simulink model "modi1_4"  (R2022b)
settings: Solver=VariableStepAuto  StartTime=0.0  StopTime=100.0  RelTol=1e-3
values from neighbouring files (symbols this model uses):
  a0 = 0.00447127    [modi1.m]
  a1 = 0.108205    [modi1.m]
  a2 = 0.683702    [modi1.m]
  alfa1 = 1.2    [modi1.m]
  alfa2 = 0.56    [modi1.m]
  alfa3 = -1.45    [modi1.m]
  alfa4 = 1.15    [modi1.m]
  b0 = 0.00201207    [modi1.m]
settings Model: Creator=zalew  LastModifiedBy=zalew

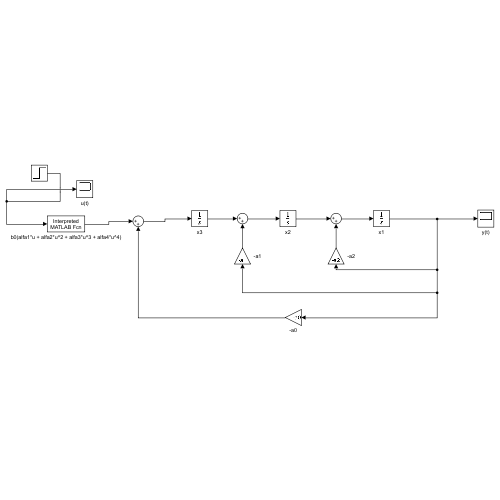
[thumbnail: Simulink's stored preview of the top-level diagram]
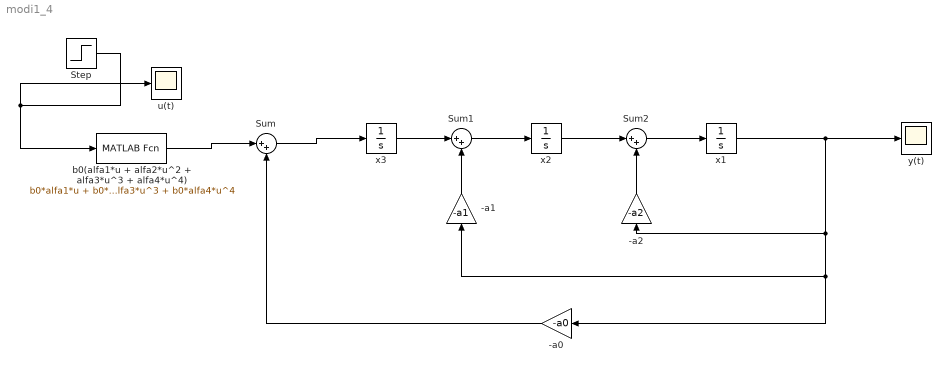
== system modi1_4 ==
  -a0 : Gain  Gain=-a0
  -a1 : Gain  Gain=-a1
  -a2 : Gain  Gain=-a2
  Step : Step  Time=10  After=0.5  SampleTime=0
  Sum : Sum  Inputs=|++
  Sum1 : Sum  Inputs=|++
  Sum2 : Sum  Inputs=|++
  b0(alfa1*u + alfa2*u^2 + alfa3*u^3 + alfa4*u^4) : MATLABFcn  MATLABFcn=b0*alfa1*u + b0*alfa2*u^2 + b0*alfa3*u^3 + b0*alfa4*u^4
  u(t) : Scope
  x1 : Integrator
  x2 : Integrator
  x3 : Integrator
  y(t) : Scope
  wires:
  b0(alfa1*u + alfa2*u^2 + alfa3*u^3 + alfa4*u^4)/1 -> Sum/1
  Sum/1 -> x3/1
  x3/1 -> Sum1/1
  Sum1/1 -> x2/1
  x2/1 -> Sum2/1
  Sum2/1 -> x1/1
  x1/1 -> y(t)/1, -a2/1, -a1/1, -a0/1
  -a0/1 -> Sum/2
  -a2/1 -> Sum2/2
  -a1/1 -> Sum1/2
  Step/1 -> u(t)/1, b0(alfa1*u + alfa2*u^2 + alfa3*u^3 + alfa4*u^4)/1
